simulink model "band_4"  (Simulink 7.8)
settings: Solver=ode45  StartTime=0.0  StopTime=1  RelTol=1e-3
values from neighbouring files (symbols this model uses):
  fc = 0.2    [TP_fdesign1.m]    (also in TP_fdesign2.m; band4.m = 2000)
  h0 = zeros(1,L)    [G722_1.m]    (also in audio_test1.m = han(:,1); audio_test2.m = han(:,1); band4.m = fir1(nf, 2*ftp))
  hbp = h0.*exp(j*2*pi*fc*(-nf/2:nf/2)/fs)    [band4.m]
  Ts = 1/fs    (= 6.25e-05)    [G722_1.m]    (also in adaptiv_2.m = 0.001; adaptiv_3.m = 0.001; adaptiv_4.m = 0.001; adaptiv_5.m = 0.001)
undefined symbols (not defined in the file or in its folder): Fs, get, sided, Two
libraries: dspsnks4 x2, dspsrcs4 x1
settings Model: Creator=svenhoffmann  LastModifiedBy=josef  ExtModeAutoUpdateStatusClock=off
settings DataIOCC: SignalLoggingName=sigsOut
settings OptimizationCC: InitFltsAndDblsToZero=on
settings DebuggingCC: SaveWithParameterizedLinksMsg=none  SignalResolutionControl=TryResolveAllWithWarning  SolverPrmCheckMsg=none  MultiTaskDSMMsg=warning  MultiTaskCondExecSysMsg=none  FcnCallInpInsideContextMsg=Use local settings  StrictBusMsg=None
settings HardwareCC: TargetUnknown=on
settings RTWCC: IncludeERTFirstTime=on
settings GRTTargetCC: TargetFcnLib=ansi_tfl_tmw.mat

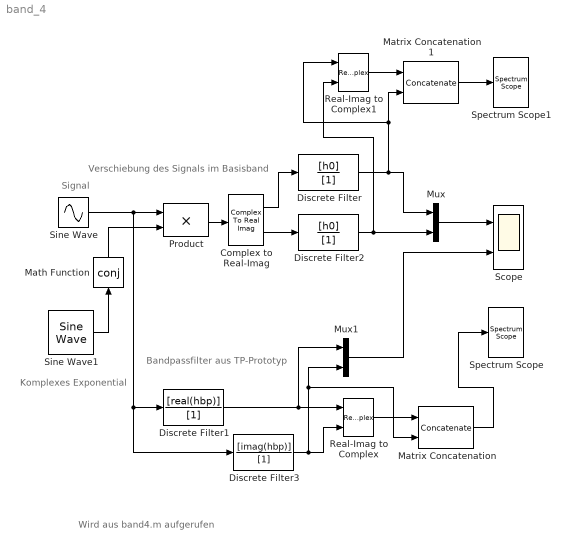
== system band_4 ==
  note: Signal
  note: Komplexes Exponential
  note: Verschiebung  des Signals
      | im Basisband
  note: Bandpassfilter
      | aus TP-Prototyp
  note: Wird aus band4.m aufgerufen
  Complex to Real-Imag : ComplexToRealImag
  Discrete Filter : DiscreteFilter  Numerator=[h0]  Denominator=[1]  SampleTime=Ts
  Discrete Filter1 : DiscreteFilter  Numerator=[real(hbp)]  Denominator=[1]  SampleTime=Ts
  Discrete Filter2 : DiscreteFilter  Numerator=[h0]  Denominator=[1]  SampleTime=Ts
  Discrete Filter3 : DiscreteFilter  Numerator=[imag(hbp)]  Denominator=[1]  SampleTime=Ts
  Math Function : Math  Operator=conj  SaturateOnIntegerOverflow=on
  Matrix Concatenation : Concatenate  Mode=Multidimensional array  ConcatenateDimension=2
  Matrix Concatenation1 : Concatenate  Mode=Multidimensional array  ConcatenateDimension=2
  Mux : Mux  Inputs=2
  Mux1 : Mux  Inputs=2
  Product : Product  SaturateOnIntegerOverflow=on  OutDataTypeStr=Inherit: Same as first input
  Real-Imag to Complex : RealImagToComplex
  Real-Imag to Complex1 : RealImagToComplex
  Scope : Scope  NumInputPorts=2
      settings: YMin=-5~-5  YMax=5~5
  Sine Wave : Sin  Frequency=2*pi*(fc+450)  SampleTime=Ts
  Sine Wave1 : dspsrcs4/Sine Wave  Amplitude=1  Frequency=fc  Phase=0  SampleMode=Discrete  OutComplex=Complex  CompMethod=Trigonometric fcn  TableSize=Speed  SampleTime=Ts  SamplesPerFrame=1  ResetState=Restart at time zero  dataType=double  wordLen=16  udDataType=sfix(16)  fracBitsMode=Best precision  numFracBits=15  OutDataTypeStr=double  LastOutDataTypeStr=double
      settings: additionalParams=on
  Spectrum Scope : dspsnks4/Spectrum Scope  ScopeProperties=on  Domain=Frequency  HorizSpan=1  UseBuffer=on  BufferSize=512  Overlap=0  TreatMby1Signals=M channels  inpFftLenInherit=off  FFTlength=128  numAvg=10  DisplayProperties=off  AxisGrid=on  Memory=off  FrameNumber=on  AxisLegend=off  AxisZoom=off  OpenScopeAtSimStart=on  OpenScopeImmediately=off  FigPos=get(0,'defaultfigureposition')  AxisProperties=off  XUnits=Hertz  XRange=Two-sided ((-Fs/2...Fs/2])  XDisplay=0  InheritXIncr=on  XIncr=1.0  XLabel=Samples  XLimit=Auto  YUnits=dBW/Hertz  XMax=1  XMin=0  YLabel=Magnitude, dB  LineProperties=off  wintypeSpecScope=Hann  RsSpecScope=50  betaSpecScope=5  winsampSpecScope=Periodic  XAxisParamsVer=6.8  isFrameUpgraded=on
      settings: YMin=-164.362377632534  YMax=13.9419115165123
  Spectrum Scope1 : dspsnks4/Spectrum Scope  ScopeProperties=off  Domain=Frequency  HorizSpan=1  UseBuffer=on  BufferSize=512  Overlap=0  TreatMby1Signals=M channels  inpFftLenInherit=off  FFTlength=128  numAvg=2  DisplayProperties=off  AxisGrid=on  Memory=off  FrameNumber=on  AxisLegend=off  AxisZoom=off  OpenScopeAtSimStart=on  OpenScopeImmediately=off  FigPos=get(0,'defaultfigureposition')  AxisProperties=on  XUnits=Hertz  XRange=Two-sided ((-Fs/2...Fs/2])  XDisplay=0  InheritXIncr=on  XIncr=-1  XLabel=Samples  XLimit=Auto  YUnits=dBW/Hertz  XMax=1  XMin=0  YLabel=Magnitude, dB  LineProperties=off  wintypeSpecScope=Hann  RsSpecScope=50  betaSpecScope=5  winsampSpecScope=Periodic  XAxisParamsVer=6.8  isFrameUpgraded=on
      settings: YMin=-156.944479149636  YMax=13.7852312029979
  wires:
  Sine Wave/1 -> Product/1, Discrete Filter1/1, Discrete Filter3/1
  Sine Wave1/1 -> Math Function/1
  Product/1 -> Complex to Real-Imag/1
  Complex to Real-Imag/1 -> Discrete Filter/1
  Complex to Real-Imag/2 -> Discrete Filter2/1
  Discrete Filter/1 -> Mux/1, Real-Imag to Complex1/1, Matrix Concatenation1/2
  Discrete Filter2/1 -> Mux/2, Real-Imag to Complex1/2
  Mux/1 -> Scope/1
  Mux1/1 -> Scope/2
  Discrete Filter1/1 -> Real-Imag to Complex/1, Mux1/1
  Discrete Filter3/1 -> Real-Imag to Complex/2, Mux1/2, Matrix Concatenation/2
  Math Function/1 -> Product/2
  Real-Imag to Complex/1 -> Matrix Concatenation/1
  Matrix Concatenation/1 -> Spectrum Scope/1
  Real-Imag to Complex1/1 -> Matrix Concatenation1/1
  Matrix Concatenation1/1 -> Spectrum Scope1/1
